simulink model "Final_Project_Fix"  (R2021a)
settings: Solver=VariableStepAuto  StartTime=0.0  StopTime=10  MaxStep=1e-3  RelTol=1e-3
settings Model: Creator=Admin  LastModifiedBy=Admin

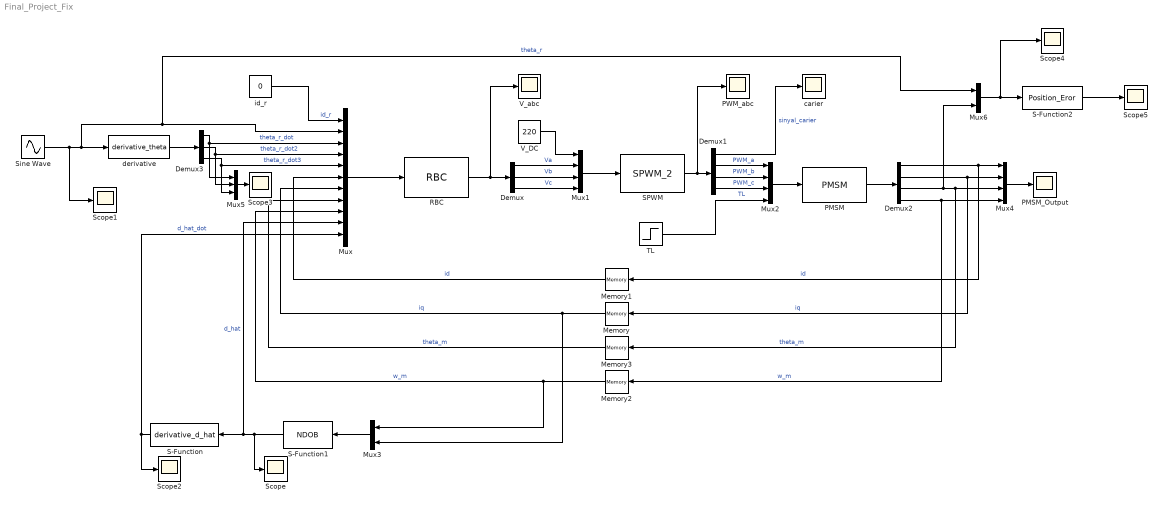
== system Final_Project_Fix ==
  Demux : Demux  Outputs=3
  Demux1 : Demux
  Demux2 : Demux
  Demux3 : Demux  Outputs=3
  Memory{,1..3} (4 alike) : Memory
  Mux : Mux  Inputs=11
  Mux1 : Mux
  Mux2 : Mux
  Mux3 : Mux  Inputs=2
  Mux4 : Mux
  Mux5 : Mux  Inputs=3
  Mux6 : Mux  Inputs=2
  PMSM : S-Function  FunctionName=PMSM  SFunctionDeploymentMode=off  EnableBusSupport=off
  PMSM_Output : Scope
  PWM_abc : Scope
  RBC : S-Function  FunctionName=RBC  SFunctionDeploymentMode=off  EnableBusSupport=off
  S-Function : S-Function  FunctionName=derivative_d_hat  SFunctionDeploymentMode=off  EnableBusSupport=off
  S-Function1 : S-Function  FunctionName=NDOB  SFunctionDeploymentMode=off  EnableBusSupport=off
  S-Function2 : S-Function  FunctionName=Position_Eror  SFunctionDeploymentMode=off  EnableBusSupport=off
  SPWM : S-Function  FunctionName=SPWM_2  SFunctionDeploymentMode=off  EnableBusSupport=off
  Scope{,1..5} (6 alike) : Scope
  Sine Wave : Sin  Amplitude=3  SampleTime=0
  TL : Step  Time=1.5  SampleTime=0
  V_DC : Constant  Value=220
  V_abc : Scope
  carier : Scope
  derivative : S-Function  FunctionName=derivative_theta  SFunctionDeploymentMode=off  EnableBusSupport=off
  id_r : Constant  Value=0
  wires:
  Mux/1 -> RBC/1
  RBC/1 -> V_abc/1, Demux/1
  Demux/1 -> Mux1/2  "Va"
  Demux/2 -> Mux1/3  "Vb"
  Demux/3 -> Mux1/4  "Vc"
  V_DC/1 -> Mux1/1
  Mux1/1 -> SPWM/1
  Mux2/1 -> PMSM/1
  PMSM/1 -> Demux2/1
  Mux3/1 -> S-Function1/1
  Demux2/1 -> Mux4/1, Memory1/1  "id"
  Demux2/2 -> Mux4/2, Memory/1  "iq"
  Demux2/3 -> Mux6/2, Mux4/3, Memory3/1  "theta_m"
  Demux2/4 -> Mux4/4, Memory2/1  "w_m"
  Memory1/1 -> Mux/6  "id"
  Memory/1 -> Mux/7, Mux3/2  "iq"
  Memory3/1 -> Mux/8  "theta_m"
  Memory2/1 -> Mux3/1, Mux/9  "w_m"
  S-Function1/1 -> Scope/1, S-Function/1, Mux/10  "d_hat"
  SPWM/1 -> PWM_abc/1, Demux1/1
  Demux1/2 -> Mux2/1  "PWM_a"
  Demux1/3 -> Mux2/2  "PWM_b"
  Demux1/4 -> Mux2/3  "PWM_c"
  Demux1/1 -> carier/1  "sinyal_carier"
  derivative/1 -> Demux3/1
  Demux3/1 -> Mux5/1, Mux/3  "theta_r_dot"
  Demux3/2 -> Mux5/2, Mux/4  "theta_r_dot2"
  Demux3/3 -> Mux5/3, Mux/5  "theta_r_dot3"
  id_r/1 -> Mux/1  "id_r"
  S-Function/1 -> Scope2/1, Mux/11  "d_hat_dot"
  TL/1 -> Mux2/4  "TL"
  Sine Wave/1 -> Scope1/1, Mux6/1, Mux/2, derivative/1  "theta_r"
  Mux4/1 -> PMSM_Output/1
  Mux5/1 -> Scope3/1
  Mux6/1 -> Scope4/1, S-Function2/1
  S-Function2/1 -> Scope5/1
